simulink model "PMSM_Control_Using_FOC_And_SVPWM"  (R2023b)
(part 2 of 3)

  PWM Generator (DC-DC)14/1 -> Mosfet16/1, NOT7/1
  NOT7/1 -> Mosfet17/1
  Constant51/1 -> PWM Generator (DC-DC)14/1
  NOT6/1 -> Mosfet13/1
  PID Controller39/1 -> PWM Generator (DC-DC)8/1
  PWM Generator (DC-DC)2/1 -> Mosfet3/1
  PWM Generator (DC-DC)3/1 -> Mosfet2/1
  Bus Selector25/2 -> Scope52/2, Scope44/2  "<Current (A)>"
  Voltage Measurement25/1 -> Display37/1
  Battery15/1 -> Bus Selector25/1
  Bus Selector25/3 -> Goto2/1, Scope52/3  "<Voltage (V)>"
  Bus Selector25/1 -> Scope44/1, Goto1/1, Scope52/1, Goto/1  "<SOC (%)>"
  From2/1 -> Mosfet22/1
  From3/1 -> Mosfet23/1
  Voltage Measurement27/1 -> Display38/1, Goto3/1
  Sum43/1 -> PID Controller43/1
  Constant53/1 -> Sum43/1
  From4/1 -> Sum43/2
  PID Controller43/1 -> Goto4/1
  PID Controller44/1 -> Gain33/1
  From5/1 -> Sum46/2
  Constant54/1 -> Sum46/1
  Sum46/1 -> PID Controller44/1
  Gain33/1 -> Goto5/1
  From6/1 -> Switch3/1
  From7/1 -> Switch3/3
  From8/1 -> Switch3/2
  Step10/1 -> Goto6/1
  From9/1 -> Ideal Switch/1
  From10/1 -> Sum47/2
  From11/1 -> Sum47/1
  Sum47/1 -> PID Controller46/1
  Switch3/1 -> Goto8/1
  PID Controller46/1 -> PWM Generator (DC-DC)16/1
  PWM Generator (DC-DC)16/1 -> NOT9/1, Goto7/1
  NOT9/1 -> Goto9/1
  From13/1 -> Mosfet19/1
  From12/1 -> Mosfet18/1
  Bus Selector26/1 -> Goto10/1, Scope54/1, Goto11/1, Scope53/1  "<SOC (%)>"
  Bus Selector26/3 -> Scope54/3, Goto12/1  "<Voltage (V)>"
  Bus Selector26/2 -> Scope53/2, Scope54/2  "<Current (A)>"
  Battery16/1 -> Bus Selector26/1
  Current Measurement9/1 -> Display40/1, Goto13/1
  NOT3/1 -> Goto15/1
  PWM Generator (DC-DC)10/1 -> Goto14/1, NOT3/1
  PID Controller47/1 -> Display41/1, PWM Generator (DC-DC)10/1
  Sum48/1 -> PID Controller47/1
  Constant46/1 -> Sum48/1
  From14/1 -> Sum48/2
  Voltage Measurement26/1 -> Display36/1
  Voltage Measurement28/1 -> Display39/1
  Signal Builder11/1(torque) -> Multiport Switch/2
  Torque_Input/1(torque) -> PMSM AC  12/1
  Battery17/1 -> Bus Selector28/1
  Bus Selector27/2 -> Subsystem/3(<Stator current is_b (A)>), Scope55/5  "<Stator current is_b (A)>"
  PMSM AC  12/1 -> Bus Selector27/1
  Bus Selector27/4 -> Subsystem/2(<Rotor speed wm (rad/s)>), Gain36/1  "<Rotor speed wm (rad/s)>"
  Bus Selector27/1 -> Scope55/4, Subsystem/1(<Stator current is_a (A)>)  "<Stator current is_a (A)>"
  Bus Selector27/3 -> Subsystem/4(<Stator current is_c (A)>), Scope55/6  "<Stator current is_c (A)>"
  Gain36/1 -> Scope55/1
  Bus Selector28/1 -> Scope59/1  "<SOC (%)>"
  Bus Selector28/3 -> Scope59/3  "<Voltage (V)>"
  Bus Selector27/6 -> Scope55/2  "<Electromagnetic torque Te (N*m)>"
  Bus Selector28/2 -> Scope59/2  "<Current (A)>"
  Bus Selector27/5 -> Subsystem/5(<Rotor angle thetam (rad)>), Scope55/3  "<Rotor angle thetam (rad)>"
  Speed_Ref/1(speed) -> Subsystem/6(Speed_Ref)
  Subsystem/1(Gates) -> Full_Bridge/1(g)
  PMSM AC  14/1 -> Bus Selector31/1
  Bus Selector31/2 -> Subsystem1/3(<Stator current is_b (A)>), Scope56/5  "<Stator current is_b (A)>"
  Bus Selector32/2 -> Scope57/2  "<Current (A)>"
  Bus Selector31/4 -> Subsystem1/2(<Rotor speed wm (rad/s)>), Gain34/1  "<Rotor speed wm (rad/s)>"
  Bus Selector31/5 -> Subsystem1/5(<Rotor angle thetam (rad)>), Scope56/3  "<Rotor angle thetam (rad)>"
  Bus Selector31/6 -> Scope56/2  "<Electromagnetic torque Te (N*m)>"
  Gain34/1 -> Scope56/1
  Battery19/1 -> Bus Selector32/1
  Recovered_Energy_Calculation/1(Output) -> Display42/1
  Torque_Input1/1(torque) -> PMSM AC  14/1
  Subsystem1/1(Gates) -> Full_Bridge1/1(g)
  Bus Selector31/3 -> Subsystem1/4(<Stator current is_c (A)>), Scope56/6  "<Stator current is_c (A)>"
  Speed_Ref1/1(speed) -> Subsystem1/6(Speed_Ref)
  Voltage Measurement29/1 -> Recovered_Energy_Calculation/2(In2)
  Current Measurement11/1 -> Recovered_Energy_Calculation/1(In1)
  Bus Selector32/3 -> Scope57/3  "<Voltage (V)>"
  Bus Selector32/1 -> Scope57/1  "<SOC (%)>"
  Bus Selector31/1 -> Scope56/4, Subsystem1/1(<Stator current is_a (A)>)  "<Stator current is_a (A)>"
  Demux26/3 -> Terminator25/1
  Alpha-Beta-Zero to dq12/1 -> Demux26/1
  Sum55/1 -> PID Controller52/1
  SVPWM Generator (2-Level)13/1 -> Universal Bridge13/1
  Bus Selector30/3 -> Scope64/3  "<Voltage (V)>"
  Sum53/1 -> Scope61/2, PID Controller53/1
  Speed_Path12/1(speed) -> Sum55/1
  Constant58/1 -> Mux25/3
  dq0 to Alpha-Beta-Zero12/1 -> Demux25/1
  PID Controller52/1 -> Scope61/1, Sum54/1
  Gain38/1 -> Sum55/2
  Bus Selector29/2 -> Scope60/5, Mux26/2  "<Stator current is_b (A)>"
  PID Controller54/1 -> Mux25/2
  Gain37/1 -> Alpha-Beta-Zero to dq12/2, dq0 to Alpha-Beta-Zero12/2
  Current Measurement13/1 -> Scope62/1, Switch4/3, Product/2
  Bus Selector30/1 -> Scope64/1  "<SOC (%)>"
  Battery18/1 -> Bus Selector30/1
  Sum54/1 -> PID Controller54/1
  Bus Selector29/6 -> Scope60/2  "<Electromagnetic torque Te (N*m)>"
  Demux25/2 -> SVPWM Generator (2-Level)13/2
  Integrator/1 -> J to Wh/1
  Demux25/3 -> Terminator24/1
  Voltage Measurement33/1 -> Product/1, Display45/1
  Bus Selector29/5 -> Scope60/3, Gain37/1  "<Rotor angle thetam (rad)>"
  Switch4/1 -> Integrator/1
  Constant59/1 -> Switch4/1
  Bus Selector30/2 -> Scope64/2  "<Current (A)>"
  Gain39/1 -> Scope60/1
  Constant57/1 -> Sum53/1
  Demux25/1 -> SVPWM Generator (2-Level)13/1
  PID Controller53/1 -> Mux25/1
  Demux26/1 -> Sum53/2
  Signal Builder13/1(torque) -> PMSM AC  13/1
  PMSM AC  13/1 -> Bus Selector29/1
  Demux26/2 -> Sum54/2
  Bus Selector29/1 -> Scope60/4, Mux26/1  "<Stator current is_a (A)>"
  abc to Alpha-Beta-Zero12/1 -> Alpha-Beta-Zero to dq12/1
  Mux25/1 -> dq0 to Alpha-Beta-Zero12/1
  Bus Selector29/4 -> Gain39/1, Gain38/1  "<Rotor speed wm (rad/s)>"
  Mux26/1 -> abc to Alpha-Beta-Zero12/1
  Bus Selector29/3 -> Scope60/6, Mux26/3  "<Stator current is_c (A)>"
  Product/1 -> Switch4/2
  J to Wh/1 -> Display46/1, Scope63/1
  Recovered_Energy_Calculation_/1(Output) -> Display43/1
  Current Measurement12/1 -> Recovered_Energy_Calculation_/1(In1)
  Voltage Measurement30/1 -> Recovered_Energy_Calculation_/2(In2)
  connections:
  DC Voltage5/LConn1 -- Universal Bridge5/RConn2
  DC Voltage5/RConn1 -- Universal Bridge5/RConn1
  Universal Bridge5/LConn1 -- PMSM AC  2/LConn1
  Universal Bridge5/LConn2 -- PMSM AC  2/LConn2
  Universal Bridge5/LConn3 -- PMSM AC  2/LConn3
  Series RLC Branch1/RConn1 -- Voltage Measurement/LConn1 -- Battery1/LConn1 -- Series RLC Branch/LConn1
  Series RLC Branch1/LConn1 -- Mosfet/LConn1 -- Mosfet1/RConn1
  Series RLC Branch/RConn1 -- Battery1/LConn2 -- Voltage Measurement/LConn2 -- Battery2/LConn2 -- Voltage Measurement1/LConn2 -- Series RLC Branch2/RConn1 -- Mosfet/RConn1
  Series RLC Branch2/LConn1 -- Battery2/LConn1 -- Voltage Measurement1/LConn1 -- Mosfet1/LConn1
  Universal Bridge1/LConn2 -- Three-Phase V-I Measurement/LConn2
  Voltage Measurement2/LConn1 -- Current Measurement/RConn1 -- Universal Bridge1/RConn1
  Universal Bridge1/LConn1 -- Three-Phase V-I Measurement/LConn1
  Voltage Measurement2/LConn2 -- Battery3/LConn2 -- Universal Bridge1/RConn2
  Universal Bridge1/LConn3 -- Three-Phase V-I Measurement/LConn3
  Mosfet2/RConn1 -- Battery5/LConn2 -- Voltage Measurement4/LConn2 -- Series RLC Branch3/RConn1 -- Universal Bridge2/RConn2 -- Voltage Measurement3/LConn2 -- Voltage Measurement5/LConn2 -- Series RLC Branch5/RConn1
  Universal Bridge2/LConn3 -- PMSM AC  3/LConn3
  Universal Bridge2/LConn1 -- PMSM AC  3/LConn1
  Universal Bridge2/LConn2 -- PMSM AC  3/LConn2
  Series RLC Branch4/RConn1 -- Voltage Measurement4/LConn1 -- Battery5/LConn1 -- Series RLC Branch3/LConn1
  Series RLC Branch4/LConn1 -- Mosfet3/LConn1 -- Mosfet2/LConn1
  Voltage Measurement3/LConn1 -- Mosfet3/RConn1 -- Series RLC Branch5/LConn1 -- Voltage Measurement5/LConn1 -- Universal Bridge2/RConn1
  Current Measurement/LConn1 -- Battery3/LConn1
  Three-Phase V-I Measurement/RConn1 -- PMSM AC  1/LConn1
  Three-Phase V-I Measurement/RConn2 -- PMSM AC  1/LConn2
  Three-Phase V-I Measurement/RConn3 -- PMSM AC  1/LConn3
  Voltage Measurement6/LConn2 -- Universal Bridge3/RConn2 -- Battery4/LConn2
  Voltage Measurement6/LConn1 -- Battery4/LConn1 -- Universal Bridge3/RConn1
  Universal Bridge3/LConn3 -- PMSM AC  4/LConn3
  Universal Bridge3/LConn2 -- PMSM AC  4/LConn2
  Universal Bridge3/LConn1 -- PMSM AC  4/LConn1
  Universal Bridge4/LConn2 -- PMSM AC  5/LConn2
  Universal Bridge4/LConn1 -- PMSM AC  5/LConn1
  Universal Bridge4/RConn2 -- Battery6/LConn2 -- Series RLC Branch6/RConn1 -- Voltage Measurement7/LConn2
  Universal Bridge4/LConn3 -- PMSM AC  5/LConn3
  Voltage Measurement7/LConn1 -- Current Measurement1/RConn1 -- Universal Bridge4/RConn1
  Current Measurement1/LConn1 -- Battery6/LConn1 -- Series RLC Branch6/LConn1
  Series RLC Branch7/RConn1 -- Battery9/LConn2 -- Voltage Measurement10/LConn2 -- Series RLC Branch11/RConn1 -- Battery10/LConn2 -- Voltage Measurement11/LConn2 -- Mosfet6/RConn1
  Voltage Measurement11/LConn1 -- Battery10/LConn1 -- Series RLC Branch11/LConn1 -- Mosfet7/LConn1
  Series RLC Branch10/LConn1 -- Mosfet7/RConn1 -- Mosfet6/LConn1
  Series RLC Branch7/LConn1 -- Series RLC Branch10/RConn1 -- Voltage Measurement10/LConn1 -- Battery9/LConn1
  Universal Bridge6/LConn2 -- PMSM AC  6/LConn2
  Universal Bridge6/LConn1 -- PMSM AC  6/LConn1
  DC Voltage1/LConn1 -- Universal Bridge6/RConn2
  Universal Bridge6/LConn3 -- PMSM AC  6/LConn3
  DC Voltage1/RConn1 -- Universal Bridge6/RConn1
  Universal Bridge7/LConn2 -- PMSM AC  7/LConn2
  Universal Bridge7/LConn1 -- PMSM AC  7/LConn1
  Universal Bridge7/RConn2 -- Battery7/LConn2 -- Series RLC Branch8/RConn1
  Universal Bridge7/LConn3 -- PMSM AC  7/LConn3
  Universal Bridge7/RConn1 -- Battery7/LConn1 -- Series RLC Branch8/LConn1
  Voltage Measurement12/LConn2 -- Mosfet5/RConn1 -- Series RLC Branch9/RConn1 -- Voltage Measurement8/LConn2 -- Universal Bridge8/RConn2 -- Voltage Measurement9/LConn2 -- Series RLC Branch14/RConn1 -- Battery11/LConn2
  Voltage Measurement8/LConn1 -- Current Measurement2/RConn1 -- Universal Bridge8/RConn1
  Universal Bridge8/LConn2 -- PMSM AC  8/LConn2
  Universal Bridge8/LConn1 -- PMSM AC  8/LConn1
  Universal Bridge8/LConn3 -- PMSM AC  8/LConn3
  Mosfet4/RConn1 -- Series RLC Branch12/LConn1 -- Mosfet5/LConn1
  Voltage Measurement12/LConn1 -- Battery11/LConn1 -- Series RLC Branch14/LConn1 -- Mosfet4/LConn1
  Voltage Measurement9/LConn1 -- Current Measurement2/LConn1 -- Series RLC Branch9/LConn1 -- Current Measurement3/RConn1
  Current Measurement3/LConn1 -- Series RLC Branch12/RConn1
  Current Measurement5/RConn1 -- Voltage Measurement15/LConn1 -- Current Measurement4/LConn1 -- Series RLC Branch16/LConn1
  Universal Bridge9/RConn2 -- Mosfet9/RConn1 -- Voltage Measurement13/LConn2 -- Battery8/LConn2 -- Series RLC Branch15/RConn1 -- Voltage Measurement15/LConn2 -- Series RLC Branch16/RConn1 -- Voltage Measurement14/LConn2
  Mosfet8/LConn1 -- Voltage Measurement13/LConn1 -- Battery8/LConn1 -- Series RLC Branch15/LConn1
  Universal Bridge9/RConn1 -- Current Measurement4/RConn1 -- Voltage Measurement14/LConn1
  Mosfet9/LConn1 -- Mosfet8/RConn1 -- Series RLC Branch13/LConn1
  Universal Bridge9/LConn2 -- PMSM AC  9/LConn2
  Universal Bridge9/LConn1 -- PMSM AC  9/LConn1
  Universal Bridge9/LConn3 -- PMSM AC  9/LConn3
  Current Measurement5/LConn1 -- Series RLC Branch13/RConn1
  Current Measurement7/RConn1 -- Series RLC Branch19/LConn1 -- Current Measurement6/LConn1 -- Voltage Measurement18/LConn1
  Universal Bridge10/RConn2 -- Voltage Measurement17/LConn2 -- Series RLC Branch19/RConn1 -- Voltage Measurement18/LConn2 -- Series RLC Branch18/RConn1 -- Battery12/LConn2 -- Voltage Measurement16/LConn2 -- Mosfet11/RConn1
  Mosfet10/LConn1 -- Series RLC Branch18/LConn1 -- Battery12/LConn1 -- Voltage Measurement16/LConn1
  Universal Bridge10/RConn1 -- Voltage Measurement17/LConn1 -- Current Measurement6/RConn1
  Mosfet11/LConn1 -- Series RLC Branch17/LConn1 -- Mosfet10/RConn1
  Universal Bridge10/LConn3 -- PMSM AC  10/LConn3
  Universal Bridge10/LConn1 -- PMSM AC  10/LConn1
  Universal Bridge10/LConn2 -- PMSM AC  10/LConn2
  Current Measurement7/LConn1 -- Series RLC Branch17/RConn1
  Voltage Measurement19/LConn2 -- Series RLC Branch21/RConn1 -- Battery13/LConn2 -- Mosfet17/RConn1 -- Series RLC Branch27/RConn1 -- Series RLC Branch22/RConn1 -- Voltage Measurement21/LConn2 -- Mosfet13/RConn1
  Universal Bridge11/LConn1 -- PMSM AC  11/LConn1
  Universal Bridge11/LConn3 -- PMSM AC  11/LConn3
  Universal Bridge11/LConn2 -- PMSM AC  11/LConn2
  Voltage Measurement22/LConn1 -- Battery14/LConn1 -- Current Measurement10/RConn1
  Voltage Measurement23/LConn1 -- Series RLC Branch26/LConn1 -- Mosfet15/LConn1 -- Series RLC Branch25/LConn1
  Series RLC Branch23/RConn1 -- Voltage Measurement22/LConn2 -- Battery14/LConn2 -- Voltage Measurement24/LConn2 -- Series RLC Branch26/RConn1 -- Voltage Measurement23/LConn2 -- Series RLC Branch25/RConn1 -- Mosfet14/RConn1
  Universal Bridge11/RConn1 -- Current Measurement8/RConn1 -- Voltage Measurement20/LConn1
  Series RLC Branch24/RConn1 -- Current Measurement10/LConn1 -- Series RLC Branch23/LConn1
  Voltage Measurement20/LConn2 -- Universal Bridge11/RConn2
  Series RLC Branch24/LConn1 -- Voltage Measurement24/LConn1 -- Mosfet14/LConn1 -- Mosfet15/RConn1
  Mosfet13/LConn1 -- Mosfet12/RConn1 -- Series RLC Branch20/RConn1
  Mosfet17/LConn1 -- Mosfet16/RConn1 -- Series RLC Branch20/LConn1
  Series RLC Branch21/LConn1 -- Voltage Measurement19/LConn1 -- Battery13/LConn1 -- Mosfet16/LConn1
  Voltage Measurement21/LConn1 -- Series RLC Branch27/LConn1 -- Series RLC Branch22/LConn1 -- Mosfet12/LConn1
  Battery15/LConn1 -- Series RLC Branch33/LConn1 -- Series RLC Branch32/LConn1 -- Voltage Measurement25/LConn1
  Series RLC Branch32/RConn1 -- Voltage Measurement27/LConn2 -- Series RLC Branch34/RConn1 -- DC Voltage Source/LConn1 -- Mosfet23/RConn1 -- Voltage Measurement25/LConn2 -- Battery15/LConn2
  Mosfet22/RConn1 -- Mosfet23/LConn1 -- Series RLC Branch33/RConn1
  Ideal Switch/RConn1 -- Voltage Measurement27/LConn1 -- Series RLC Branch34/LConn1 -- Mosfet22/LConn1
  DC Voltage Source/RConn1 -- Ideal Switch/LConn1
  Series RLC Branch29/LConn1 -- Current Measurement9/LConn1 -- Series RLC Branch28/LConn1
  Series RLC Branch30/RConn1 -- Voltage Measurement26/LConn2 -- Mosfet19/RConn1 -- Voltage Measurement28/LConn2 -- Battery16/LConn2 -- Series RLC Branch28/RConn1 -- Series RLC Branch31/RConn1
  Mosfet19/LConn1 -- Mosfet18/RConn1 -- Series RLC Branch29/RConn1
  Series RLC Branch30/LConn1 -- Voltage Measurement26/LConn1 -- Series RLC Branch31/LConn1 -- Mosfet18/LConn1
  Current Measurement9/RConn1 -- Voltage Measurement28/LConn1 -- Battery16/LConn1
  Full_Bridge/LConn1 -- PMSM AC  12/LConn1
  Full_Bridge/LConn2 -- PMSM AC  12/LConn2
  Full_Bridge/LConn3 -- PMSM AC  12/LConn3
  Bidirectional_Converter/RConn1 -- Full_Bridge/RConn1
  Bidirectional_Converter/RConn2 -- Full_Bridge/RConn2
  Battery19/LConn2 -- Voltage Measurement29/LConn2 -- Full_Bridge1/RConn2
  Battery19/LConn1 -- Voltage Measurement29/LConn1 -- Current Measurement11/LConn1
  Full_Bridge1/LConn1 -- PMSM AC  14/LConn1
  Full_Bridge1/LConn3 -- PMSM AC  14/LConn3
  Full_Bridge1/LConn2 -- PMSM AC  14/LConn2
  Current Measurement11/RConn1 -- Full_Bridge1/RConn1
  Universal Bridge13/RConn2 -- Series RLC Branch38/RConn1 -- Voltage Measurement33/LConn2 -- Battery18/LConn2
  Current Measurement13/RConn1 -- Series RLC Branch38/LConn1 -- Universal Bridge13/RConn1
  Battery18/LConn1 -- Current Measurement13/LConn1 -- Voltage Measurement33/LConn1
  Universal Bridge13/LConn1 -- PMSM AC  13/LConn1
  Universal Bridge13/LConn3 -- PMSM AC  13/LConn3
  Universal Bridge13/LConn2 -- PMSM AC  13/LConn2
  Current Measurement12/LConn1 -- Battery17/LConn1 -- Voltage Measurement30/LConn1
  Voltage Measurement30/LConn2 -- Bidirectional_Converter/LConn2 -- Battery17/LConn2
  Current Measurement12/RConn1 -- Bidirectional_Converter/LConn1
